simulink model "GAS_turbine_frequency"  (R2024a)
settings: Solver=VariableStepAuto  StartTime=0.0  StopTime=40  RelTol=1e-3
libraries: spsThreePhaseParallelRLCLoadLib x1, spsSynchronousMachinepuStandardLib x1, spsThreePhaseBreakerLib x1, spsExcitationSystemLib x1, spsThreePhasePISectionLineLib x1, spsThreePhaseSeriesRLCLoadLib x1, spsThreePhaseSourceLib x1, spspowerguiLib x1
settings Model: Creator=李嘉楠  LastModifiedBy=Vincent-Oracle
settings RTWCC: GPUComputeCapability=3.5

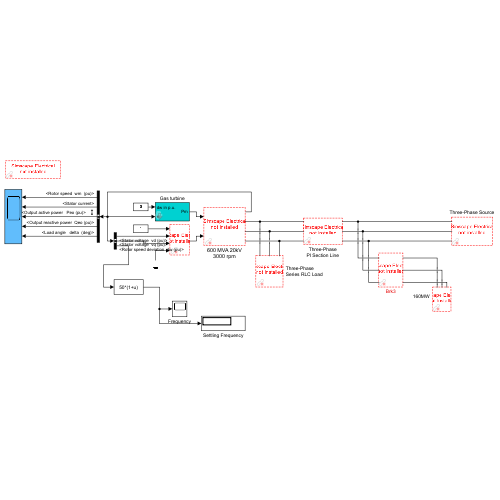
[thumbnail: Simulink's stored preview of the top-level diagram]
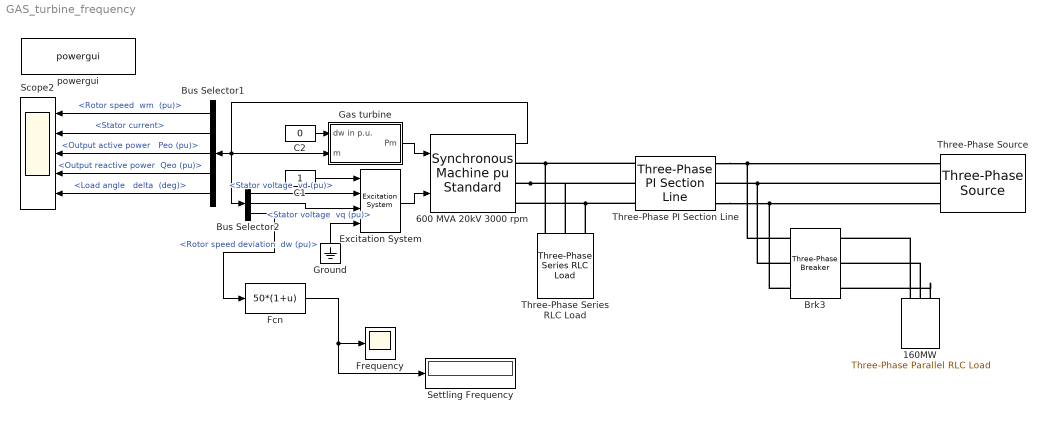
== system GAS_turbine_frequency ==
  "160MW " : spsThreePhaseParallelRLCLoadLib/Three-Phase Parallel RLC Load  LConnTagsString=A|B|C  Configuration=Y (grounded)  NominalVoltage=20E3  Vabc=[1e3 1e3 1e3]  Vabcp=[1e3 1e3 1e3]  NominalFrequency=50  UnbalancedPower=off  ActivePower=160e6  InductivePower=1E6  CapacitivePower=0  Pabc=[10e3 9e3 11e3]  QLabc=[100 90 110]  QCabc=[100 90 110]  Pabcp=[10e3 9e3 11e3]  QLabcp=[100 90 110]  QCabcp=[100 90 110]  Measurements=None  LoadType=constant PQ
  600 MVA 20kV 3000 rpm : spsSynchronousMachinepuStandardLib/Synchronous Machine pu Standard  PresetModel=No  MechanicalLoad=Mechanical power Pm  ShowDetailedParameters=on  RotorType=Round  Units=per unit standard parameters  MeasurementBus=off  NominalParameters="[100E6 20e3   50 ]"  Reactances1=[ 1.65, 0.25, 0.2, 1.59, 0.46, 0.2, 0.14 ]./1.1  Reactances2="[ 1.305, 0.296, 0.252, 0.474,  0.243,  0.18 ]"  dAxisTimeConstants=Open-circuit  qAxisTimeConstants=Open-circuit  TimeConstants1="[ 4.4849  0.0681  0.1  ]"  TimeConstants2="[ 4.5, 0.04,  0.67, 0.09 ]"  TimeConstants3="[  4.49  0.0681  0.0513  ]"  TimeConstants4=[ 8.0, 0.03, 0.3371, 0.0295 ]  TimeConstants5=[ 1.01, 0.053, 0.1 ]  TimeConstants6=[ 1.3201, 0.023, 1.0, 0.07 ]  TimeConstants7="[  1.01  0.053  0.051266  ]"  TimeConstants8=[ 1.3201, 0.0231, 0.3371, 0.0295 ]  StatorResistance=0.0045  Mechanical="[ 15.64/2  0 1 ]"  PolePairs=1  InitialConditions=[0 -109.322 5.86664e-07 5.86664e-07 5.86664e-07 -19.3222 -139.322 100.678 0.903413]  SetSaturation=off  Saturation=[0.6404,0.7127,0.8441,0.9214,0.9956,1.082,1.19,1.316,1.457;0.7,0.7698,0.8872,0.9466,0.9969,1.046,1.1,1.151,1.201]  LoadFlowParameters=[4 30.051 24 0 0]  TsPowergui=0  TsBlock=-1  IterativeModel=Trapezoidal non iterative  IterativeDiscreteModel=Trapezoidal non iterative  BusType=PQ  Pref=100E6  Qref=0  Qmin=-Inf  Qmax=Inf  PLF=0  QLF=0
  Brk3 : spsThreePhaseBreakerLib/Three-Phase Breaker  InitialState=open  SwitchA=on  SwitchB=on  SwitchC=on  SwitchTimes=[20]  External=off  BreakerResistance=0.001  SnubberResistance=inf  SnubberCapacitance=0  Measurements=None
      settings: AttributesFormatString=\n
  Bus Selector1 : BusSelector  OutputSignals="Mechanical.Rotor speed  wm  (pu),Stator current,Output active power   Peo (pu),Output reactive power  Qeo (pu),Load angle   delta  (deg)"
  Bus Selector2 : BusSelector  OutputSignals="dq0 components.Stator voltage  vd (pu),dq0 components.Stator voltage  vq (pu),Mechanical.Rotor speed deviation  dw (pu)"
  C1 : Constant
  C2 : Constant  Value=0
  Excitation System : spsExcitationSystemLib/Excitation System  tr=20e-3  reg=[ 50, 0.001 ]  exc=[ 1, 0 ]  tgr=[ 0, 0 ]  damp=[ 0.001, 0.1 ]  sat=[ 0, 0 ]  lim=[ 0 4, 0 0]  v0=[0.0012,0.903413]
      settings: LibrarySourceBlock=sps_lib/Electrical Machines/Synchronous Machine Control/Excitation System
  Fcn : Fcn  Expr=50*(1+u)
  Frequency : Scope
  Gas turbine : Subsystem  mask(Gas Turbine Regulator){T0=1, Sbase=100, W=16.7, X=0.6, Y=1, Z=1, MAX=1.5, MIN=-0.13, a=1, b=0.05, c=1, Wmin=0.23, TF=0.4, KF=0, ECR=0.01, ETD=0.04, TCD=0.2, TR=950, TT=450, TI=15.64}
      mask prompts: T0 "Initial Output Power (T0, pu)"; Sbase "Rated Generator Power (S, MVA)"; W "Speed Governor Gain (W = 1/droop, pu MW/pu speed)"; X "Speed Governor Lead Constant (X, s)"; Y "Speed Governor Lag Constant (Y, s)"; Z "Speed Governor Mode (1 = droop, 0 = isochronus)"; MAX "Fuel Demand Signal Max Limit (MAX, pu)"; MIN "Fuel Demand Signal Min Limit (MIN, pu)"; a "Valve Positioner Parameter (a)"; b "Valve Positioner Time Constant (b, s)"; c "Valve Positioner Parameter (c)"; Wmin "No Load Fuel Consumption (Wmin)"; TF "Fuel System Time Constant (TF, s)"; KF "Fuel System External Feedback Loop Gain (KF)"; ECR "Delay of Combustion System (ECR, s)"; ETD "Transport Delay of Turbine and Exhaust System (ETD, s)"; TCD "Compressor Discharge Lag Time Contant (TCD, s)"; TR "Rated Exhaust Temperature (TR, degF)"; TT "Temperature Contoller Integration Constant (TT, degF)"; TI "Inertia (TI = 2*H)"
      mask help:
      | Full Rowen's model for HDGTs for dynamic studies.
      |
      | Limits of applicability:
      | 1. For simple cycle, single-shaft, generator drive only.
      | 2. Allowable speed range = 0.95 - 1.07 of rated speed.
      | 3. No heat recovery.
      | 4. ISO conditions.
      |
      | Model created according to the papers:
      | 1. W. I. Rowen,  Simplified mathematic representations of heavy-duty gas turbines, oct. 1983, p. 865
      | 2. Mohammad Reza Bank Tavakoli, Behrooz Vahidi and Wolfgang Gawlik, An Educational Guide to Extract
      | the Parameters of Heavy Duty Gas Turbines Model in Dynamic Studies Based on Operational Data
      mask Help:
      | Full Rowen's model for HDGTs for dynamic studies.
      | 
      | Limits of applicability:
      | 1. For simple cycle, single-shaft, generator drive only.
      | 2. Allowable speed range = 0.95 - 1.07 of rated speed.
      | 3. No heat recovery.
      | 4. ISO conditions.
      | 
      | Model created according to the papers:
      | 1. W. I. Rowen,  Simplified mathematic representations of heavy-duty gas turbines, oct. 1983, p. 865
      | 2. Mohammad Reza Bank Tavakoli, Behrooz Vahidi and Wolfgang Gawlik, An Educational Guide to Extract
      | the Parameters of Heavy Duty Gas Turbines Model in Dynamic Studies Based on Operational Data
  Ground : Ground
  Scope2 : Scope  NumInputPorts=5
  Settling Frequency : Display
  Three-Phase PI Section Line : spsThreePhasePISectionLineLib/Three-Phase PI Section Line  LConnTagsString=a|b|c  RConnTagsString=A|B|C  Length=5  Frequency=50  Resistances=[ 0.01273 0.3864]  Inductances="[ 0.9337e-3  4.1264e-3]"  Capacitances=[12.74e-9 7.751e-9]
  Three-Phase Series RLC Load : spsThreePhaseSeriesRLCLoadLib/Three-Phase Series RLC Load  LConnTagsString=A|B|C  Configuration=Y (grounded)  NominalVoltage=20E3  Vabc=[1e3 1e3 1e3]  Vabcp=[1e3 1e3 1e3]  NominalFrequency=50  UnbalancedPower=off  ActivePower=100E6  InductivePower=1E6  CapacitivePower=0  Pabc=[10e3 9e3 11e3]  QLabc=[100 90 110]  QCabc=[100 90 110]  Pabcp=[10e3 9e3 11e3]  QLabcp=[100 90 110]  QCabcp=[100 90 110]  Measurements=None  LoadType=constant Z
  Three-Phase Source : spsThreePhaseSourceLib/Three-Phase Source  InternalConnection=Y  VoltagePhases=off  Voltage=20E3  PhaseAngle=0  Voltage_phases=[25e3 25e3 25e3]/sqrt(3)  PhaseAngles_phases=[0 -120 +120]  Frequency=50  NonIdealSource=on  SpecifyImpedance=off  Resistance=.1  Inductance=0  ShortCircuitLevel=100e6  BaseVoltage=20E3  XRratio=7  BusType=swing  Pref=0  Qref=0  Prefabc=[10e3, 10e3, 10e3]  Qrefabc=[0, 0, 0]  Qmin=-inf  Qmax=inf
  powergui : spspowerguiLib/powergui  Priority=2  SimulationMode=Discrete  SampleTime=50E-6  frequency=60  Iterations=50  frequencyindice=50  Pbase=100e6  ErrMax=1e-4  UnitsV=kV  UnitsW=MW  buscounter=0  FunctionMessages=off  echomessages=off  EnableUseOfTLC=off  CurrentSourceSwitches=off  DisableSnubberDevices=off  DisableRonSwitches=off  DisableVfSwitches=off  DisplayEquations=off  AutomaticDiscreteSolvers=off  SolverType=Tustin  Interpol=off  ExternalGateDelay=off  methode=off  Ts=0  x0status=blocks  SPID=off  SwTol=0  HookPort=off  NonlinearTolerance=1e-4  nMaxIteration=100  ContinueOnMaxIteration=off  RestoreLinks=warning  ResistiveCurrentMeasurement=off  Frange=logspace(0,3,50)  Ylog=off  Xlog=off  ShowGrid=off  save=off  variable=ZData  structure=VaIa  ZoomFFT=on  StartTime=0.2  cycles=2  DisplayStyle=1  fundamental=60  FreqAxis=off  MaxFrequency=1000  frequencyindicesteady=1  RmsSteady=2  display=off
  wires:
  C1/1 -> Excitation System/1
  Bus Selector2/2 -> Excitation System/3  "<Stator voltage  vq (pu)>"
  Bus Selector1/2 -> Scope2/2  "<Stator current>"
  Bus Selector1/5 -> Scope2/5  "<Load angle   delta  (deg)>"
  Bus Selector2/1 -> Excitation System/2  "<Stator voltage  vd (pu)>"
  Gas turbine/1(Pm) -> 600 MVA 20kV 3000 rpm/1
  Bus Selector1/1 -> Scope2/1  "<Rotor speed  wm  (pu)>"
  Bus Selector1/3 -> Scope2/3  "<Output active power   Peo (pu)>"
  600 MVA 20kV 3000 rpm/1 -> Gas turbine/2(m), Bus Selector1/1, Bus Selector2/1
  Excitation System/1 -> 600 MVA 20kV 3000 rpm/2
  Ground/1 -> Excitation System/4
  C2/1 -> Gas turbine/1(dw in p.u.)
  Fcn/1 -> Settling Frequency/1, Frequency/1
  Bus Selector1/4 -> Scope2/4  "<Output reactive power  Qeo (pu)>"
  Bus Selector2/3 -> Fcn/1  "<Rotor speed deviation  dw (pu)>"
  connections:
  Three-Phase PI Section Line/LConn1 -- Three-Phase Series RLC Load/LConn1 -- 600 MVA 20kV 3000 rpm/RConn1
  600 MVA 20kV 3000 rpm/RConn2 -- Three-Phase Series RLC Load/LConn2 -- Three-Phase PI Section Line/LConn2
  Three-Phase PI Section Line/LConn3 -- Three-Phase Series RLC Load/LConn3 -- 600 MVA 20kV 3000 rpm/RConn3
  Three-Phase PI Section Line/RConn3 -- Brk3/LConn3 -- Three-Phase Source/RConn3
  Three-Phase Source/RConn2 -- Brk3/LConn2 -- Three-Phase PI Section Line/RConn2
  Three-Phase PI Section Line/RConn1 -- Brk3/LConn1 -- Three-Phase Source/RConn1
  "160MW "/LConn2 -- Brk3/RConn2
  "160MW "/LConn1 -- Brk3/RConn1
  "160MW "/LConn3 -- Brk3/RConn3

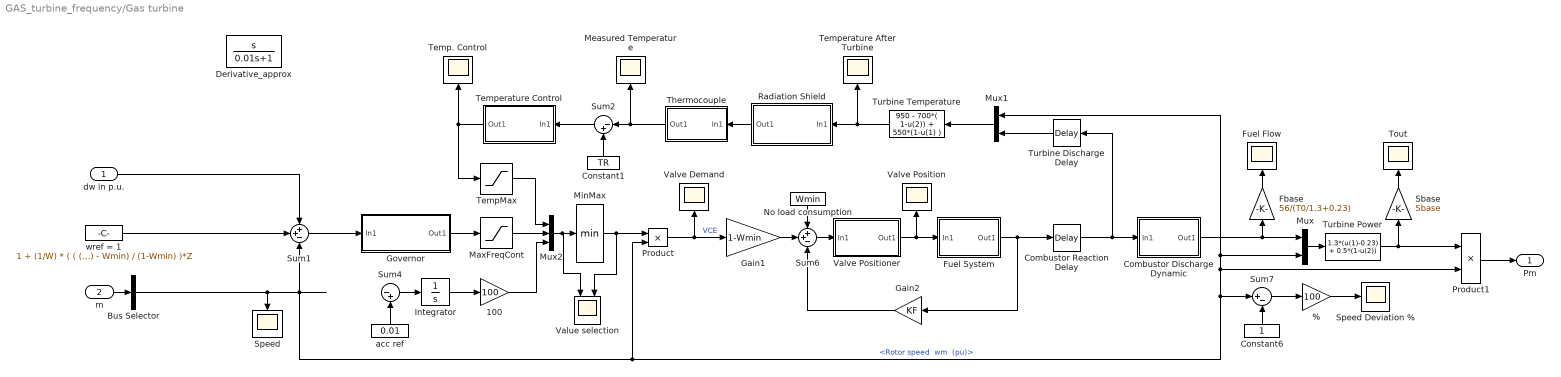
== system GAS_turbine_frequency/Gas turbine ==
  dw in p.u. : Inport
  m : Inport  Port=2
  % : Gain  Gain=100
  100 : Gain  Gain=100
  Bus Selector : BusSelector  OutputSignals="Mechanical.Rotor speed  wm  (pu)"
  Combustor Discharge Dynamic : Subsystem
      mask Display: fprintf('1/(TCD.s+1)')
  Combustor Reaction Delay : TransportDelay  DelayTime=ECR  InitialOutput=T0/1.3+0.23
  Constant1 : Constant  Value=TR
  Constant6 : Constant
  Derivative_approx : TransferFcn  Numerator=[1 0]  Denominator=[0.01 1]
  Fbase : Gain  Gain=56/(T0/1.3+0.23)
  Fuel Flow : Scope
  Fuel System : Subsystem
      mask Display: fprintf('1/(TF.s+1)')
  Gain1 : Gain  Gain=1-Wmin
  Gain2 : Gain  Gain=KF
  Governor : Subsystem
      mask Display: fprintf('W(Xs+1)/(Ys+Z)')
  Integrator : Integrator  InitialCondition=1
  MaxFreqCont : Saturate  UpperLimit=MAX  LowerLimit=MIN
  Measured Temperature : Scope
  MinMax : MinMax
  Mux : Mux  Inputs=2
  Mux1 : Mux  Inputs=2
  Mux2 : Mux  Inputs=3
  No load consumption : Constant  Value=Wmin
  Product : Product  RndMeth=Zero
  Product1 : Product  RndMeth=Zero
  Radiation Shield : Subsystem
      mask Display: fprintf('0.2/(15s+1)+0.8')
  Sbase : Gain  Gain=Sbase
  Speed : Scope
  Speed Deviation % : Scope
  Sum1 : Sum  Inputs=++-
  Sum2 : Sum  Inputs=|-+
  Sum4 : Sum  Inputs=|-+
  Sum6 : Sum  Inputs=++-
  Sum7 : Sum  Inputs=|+-
  Temp. Control : Scope
  TempMax : Saturate  UpperLimit=MAX  LowerLimit=MIN
  Temperature After Turbine : Scope
  Temperature Control : Subsystem
      mask Display: fprintf('(3.3s+1)/TT.s')
  Thermocouple : Subsystem
      mask Display: fprintf('1/(2.5s+1)')
  Tout : Scope
  Turbine Discharge Delay : TransportDelay  DelayTime=ETD  InitialOutput=T0/1.3+0.23
  Turbine Power : Fcn  Expr=1.3*(u(1)-0.23) + 0.5*(1-u(2))
  Turbine Temperature : Fcn  Expr=950 - 700*( 1-u(2)) + 550*(1-u(1) )
  Value selection : Scope  NumInputPorts=2
  Valve Demand : Scope
  Valve Position : Scope
  Valve Positioner : Subsystem
      mask Display: fprintf('a/(b.s+c)')
  acc ref : Constant  Value=0.01
  wref = 1 : Constant  Value=1 + (1/W) * ( ( (T0/1.3 + 0.23)*(c/a) - Wmin) / (1-Wmin) )*Z
  Pm : Outport
  wires:
  m/1 -> Bus Selector/1
  Bus Selector/1 -> Sum1/3, Product1/2, Mux1/1, Mux/2, Sum7/1, Product/2, Speed/1  "<Rotor speed  wm  (pu)>"
  Sum1/1 -> Governor/1(In1)
  Thermocouple/1(Out1) -> Sum2/1, Measured Temperature/1
  Constant1/1 -> Sum2/2
  Integrator/1 -> 100/1
  Sum4/1 -> Integrator/1
  ? -> Sum4/1
  acc ref/1 -> Sum4/2
  Combustor Discharge Dynamic/1(Out1) -> Mux/1, Fbase/1
  Turbine Power/1 -> Product1/1, Sbase/1
  Product/1 -> Valve Demand/1, Gain1/1  "VCE"
  Sum6/1 -> Valve Positioner/1(In1)
  Sum2/1 -> Temperature Control/1(In1)
  Valve Positioner/1(Out1) -> Fuel System/1(In1), Valve Position/1
  Fuel System/1(Out1) -> Gain2/1, Combustor Reaction Delay/1
  Combustor Reaction Delay/1 -> Combustor Discharge Dynamic/1(In1), Turbine Discharge Delay/1
  Gain2/1 -> Sum6/3
  Turbine Discharge Delay/1 -> Mux1/2
  Gain1/1 -> Sum6/2
  No load consumption/1 -> Sum6/1
  Temperature Control/1(Out1) -> Temp. Control/1, TempMax/1
  Mux/1 -> Turbine Power/1
  Governor/1(Out1) -> MaxFreqCont/1
  Constant6/1 -> Sum7/2
  Sum7/1 -> %/1
  %/1 -> Speed Deviation %/1
  Turbine Temperature/1 -> Radiation Shield/1(In1), Temperature After Turbine/1
  Mux1/1 -> Turbine Temperature/1
  Radiation Shield/1(Out1) -> Thermocouple/1(In1)
  Sbase/1 -> Tout/1
  Fbase/1 -> Fuel Flow/1
  Product1/1 -> Pm/1
  MinMax/1 -> Product/1, Value selection/2
  Mux2/1 -> Value selection/1, MinMax/1
  MaxFreqCont/1 -> Mux2/2
  100/1 -> Mux2/3
  TempMax/1 -> Mux2/1
  wref = 1/1 -> Sum1/2
  dw in p.u./1 -> Sum1/1

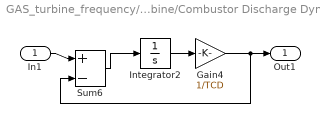
== system GAS_turbine_frequency/Gas turbine/Combustor Discharge Dynamic ==
  In1 : Inport
  Gain4 : Gain  Gain=1/TCD
  Integrator2 : Integrator  InitialCondition=TCD*(T0/1.3+0.23)
  Sum6 : Sum  Inputs=|+-
  Out1 : Outport
  wires:
  Integrator2/1 -> Gain4/1
  Gain4/1 -> Sum6/2, Out1/1
  Sum6/1 -> Integrator2/1
  In1/1 -> Sum6/1

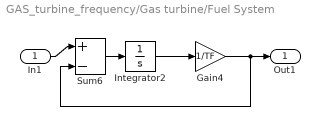
== system GAS_turbine_frequency/Gas turbine/Fuel System ==
  In1 : Inport
  Gain4 : Gain  Gain=1/TF
  Integrator2 : Integrator  InitialCondition=TF*(T0/1.3+0.23)
  Sum6 : Sum  Inputs=|+-
  Out1 : Outport
  wires:
  Integrator2/1 -> Gain4/1
  Gain4/1 -> Sum6/2, Out1/1
  Sum6/1 -> Integrator2/1
  In1/1 -> Sum6/1

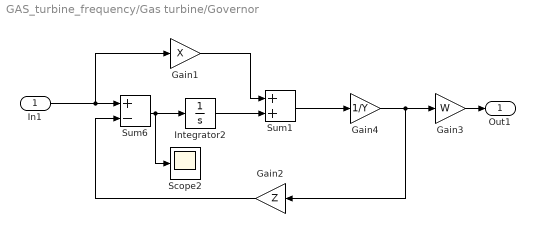
== system GAS_turbine_frequency/Gas turbine/Governor ==
  In1 : Inport
  Gain1 : Gain  Gain=X
  Gain2 : Gain  Gain=Z
  Gain3 : Gain  Gain=W
  Gain4 : Gain  Gain=1/Y
  Integrator2 : Integrator  InitialCondition=(Y-Z*X)*(1/W)*(((T0/1.3+0.23)*(c/a)-Wmin)/(1-Wmin))
  Scope2 : Scope
  Sum1 : Sum
  Sum6 : Sum  Inputs=+-
  Out1 : Outport
  wires:
  Gain4/1 -> Gain2/1, Gain3/1
  Sum6/1 -> Scope2/1, Integrator2/1
  In1/1 -> Sum6/1, Gain1/1
  Integrator2/1 -> Sum1/2
  Gain1/1 -> Sum1/1
  Gain2/1 -> Sum6/2
  Sum1/1 -> Gain4/1
  Gain3/1 -> Out1/1

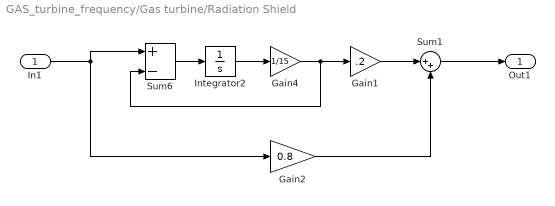
== system GAS_turbine_frequency/Gas turbine/Radiation Shield ==
  In1 : Inport
  Gain1 : Gain  Gain=.2
  Gain2 : Gain  Gain=0.8
  Gain4 : Gain  Gain=1/15
  Integrator2 : Integrator  InitialCondition=15*(950-700*(1-T0/1.3-0.23))
  Sum1 : Sum  Inputs=|++
  Sum6 : Sum  Inputs=|+-
  Out1 : Outport
  wires:
  Integrator2/1 -> Gain4/1
  Gain4/1 -> Sum6/2, Gain1/1
  Sum6/1 -> Integrator2/1
  In1/1 -> Sum6/1, Gain2/1
  Gain1/1 -> Sum1/1
  Sum1/1 -> Out1/1
  Gain2/1 -> Sum1/2

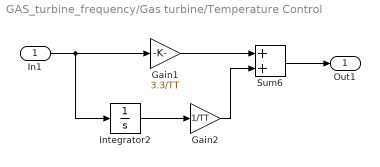
== system GAS_turbine_frequency/Gas turbine/Temperature Control ==
  In1 : Inport
  Gain1 : Gain  Gain=3.3/TT
  Gain2 : Gain  Gain=1/TT
  Integrator2 : Integrator  InitialCondition=950
  Sum6 : Sum
  Out1 : Outport
  wires:
  Sum6/1 -> Out1/1
  In1/1 -> Gain1/1, Integrator2/1
  Gain1/1 -> Sum6/1
  Integrator2/1 -> Gain2/1
  Gain2/1 -> Sum6/2

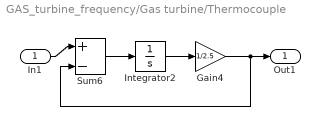
== system GAS_turbine_frequency/Gas turbine/Thermocouple ==
  In1 : Inport
  Gain4 : Gain  Gain=1/2.5
  Integrator2 : Integrator  InitialCondition=2.5*((950-700*(1-T0/1.3-0.23)))
  Sum6 : Sum  Inputs=|+-
  Out1 : Outport
  wires:
  Integrator2/1 -> Gain4/1
  Gain4/1 -> Sum6/2, Out1/1
  Sum6/1 -> Integrator2/1
  In1/1 -> Sum6/1

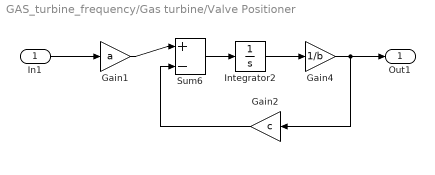
== system GAS_turbine_frequency/Gas turbine/Valve Positioner ==
  In1 : Inport
  Gain1 : Gain  Gain=a
  Gain2 : Gain  Gain=c
  Gain4 : Gain  Gain=1/b
  Integrator2 : Integrator  InitialCondition=b*(T0/1.3+0.23)
  Sum6 : Sum  Inputs=|+-
  Out1 : Outport
  wires:
  Integrator2/1 -> Gain4/1
  Gain4/1 -> Out1/1, Gain2/1
  Sum6/1 -> Integrator2/1
  In1/1 -> Gain1/1
  Gain1/1 -> Sum6/1
  Gain2/1 -> Sum6/2
